simulink model "Orbit_SRP"  (R2021b)
settings: Solver=VariableStepAuto  StartTime=0.0  StopTime=SimTime  MaxStep=1e-2  RelTol=1e-13
values from neighbouring files (symbols this model uses):
  a = 8.6251e+06    (= 8625100)    [Lab7.m]    (also in Lab_7.m = 42164; car2kep.m = -(mu/(2*E)))
  e = 0.1195    [Lab7.m]    (also in Lab_7.m = 0; car2kep.m = 1/mu * [((v_norm)^2 - (mu/r_norm)).*r - (dot(r, v).*v)])
  i = acos(h_z/h_norm)    [car2kep.m]
  mu = 398600    [Lab_7.m]
undefined symbols (not defined in the file or in its folder): A_BN, theta_0
libraries: simulink_extras x1
settings Model: Creator=adity  LastModifiedBy=adity

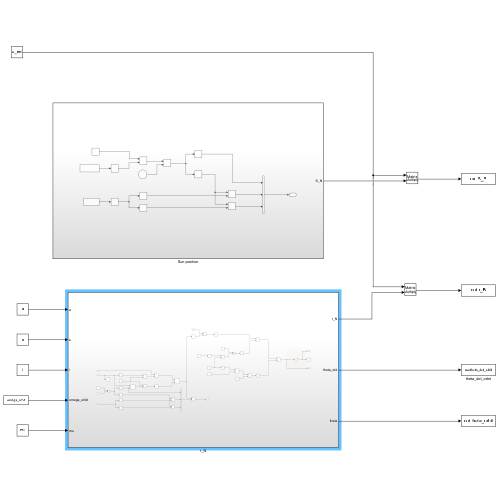
[thumbnail: Simulink's stored preview of the top-level diagram]
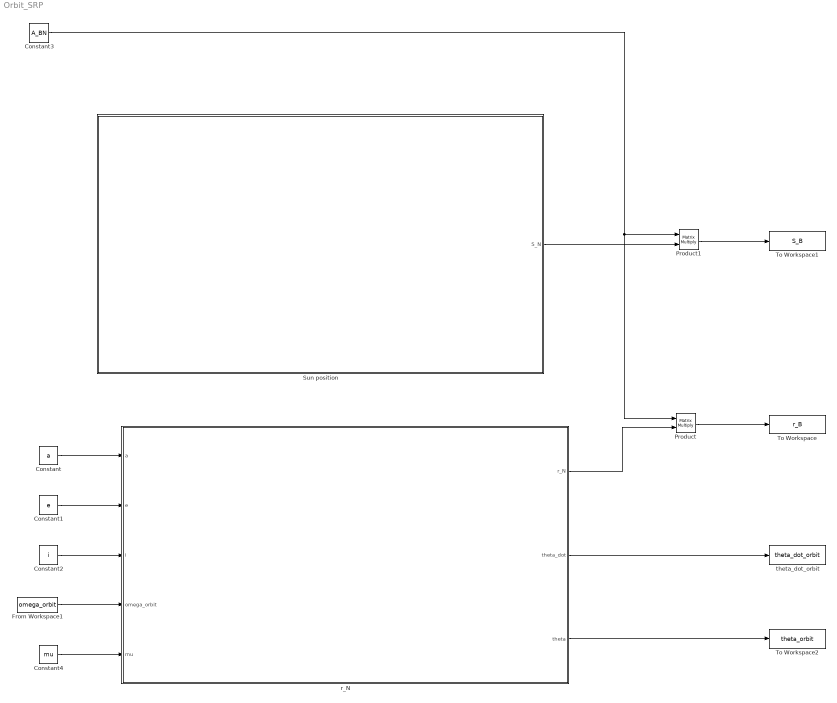
== system Orbit_SRP ==
  Constant : Constant  Value=a
  Constant1 : Constant  Value=e
  Constant2 : Constant  Value=i
  Constant3 : Constant  Value=A_BN
  Constant4 : Constant  Value=mu
  From Workspace1 : FromWorkspace  VariableName=omega_orbit
  Product : Product  Multiplication=Matrix(*)
  Product1 : Product  Multiplication=Matrix(*)
  Sun position : Subsystem
  To Workspace : ToWorkspace  VariableName=r_B  SaveFormat=Timeseries  SampleTime=-1
  To Workspace1 : ToWorkspace  VariableName=S_B  SaveFormat=Timeseries  SampleTime=-1
  To Workspace2 : ToWorkspace  VariableName=theta_orbit  SaveFormat=Timeseries  SampleTime=-1
  r_N : Subsystem
  theta_dot_orbit : ToWorkspace  VariableName=theta_dot_orbit  SaveFormat=Timeseries  SampleTime=-1
  wires:
  Constant/1 -> r_N/1(a)
  Constant1/1 -> r_N/2(e)
  Constant2/1 -> r_N/3(i)
  From Workspace1/1 -> r_N/4(omega_orbit)
  Constant4/1 -> r_N/5(mu)
  Constant3/1 -> Product/1, Product1/1
  r_N/1(r_N) -> Product/2
  Product/1 -> To Workspace/1
  r_N/2(theta_dot) -> theta_dot_orbit/1
  r_N/3(theta) -> To Workspace2/1
  Sun position/1(S_N) -> Product1/2
  Product1/1 -> To Workspace1/1

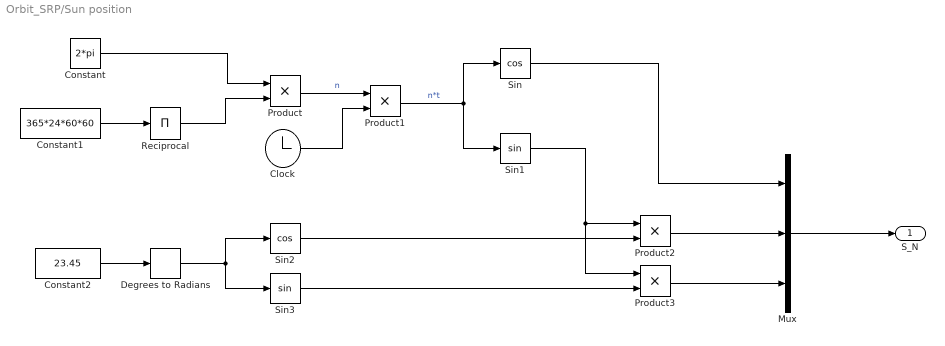
== system Orbit_SRP/Sun position ==
  Clock : Clock
  Constant : Constant  Value=2*pi
  Constant1 : Constant  Value=365*24*60*60
  Constant2 : Constant  Value=23.45
  Degrees to Radians : simulink_extras/Transformations/Degrees to Radians
  Mux : Mux  Inputs=3
  Product{,1..3} (4 alike) : Product
  Reciprocal : Product  Inputs=1
  Sin : Trigonometry  Operator=cos
  Sin1 : Trigonometry
  Sin2 : Trigonometry  Operator=cos
  Sin3 : Trigonometry
  S_N : Outport
  wires:
  Mux/1 -> S_N/1
  Constant1/1 -> Reciprocal/1
  Reciprocal/1 -> Product/2
  Constant/1 -> Product/1
  Product1/1 -> Sin/1, Sin1/1  "n*t"
  Product/1 -> Product1/1  "n"
  Clock/1 -> Product1/2
  Constant2/1 -> Degrees to Radians/1
  Sin/1 -> Mux/1
  Sin1/1 -> Product3/1, Product2/1
  Sin2/1 -> Product2/2
  Product2/1 -> Mux/2
  Sin3/1 -> Product3/2
  Product3/1 -> Mux/3
  Degrees to Radians/1 -> Sin3/1, Sin2/1

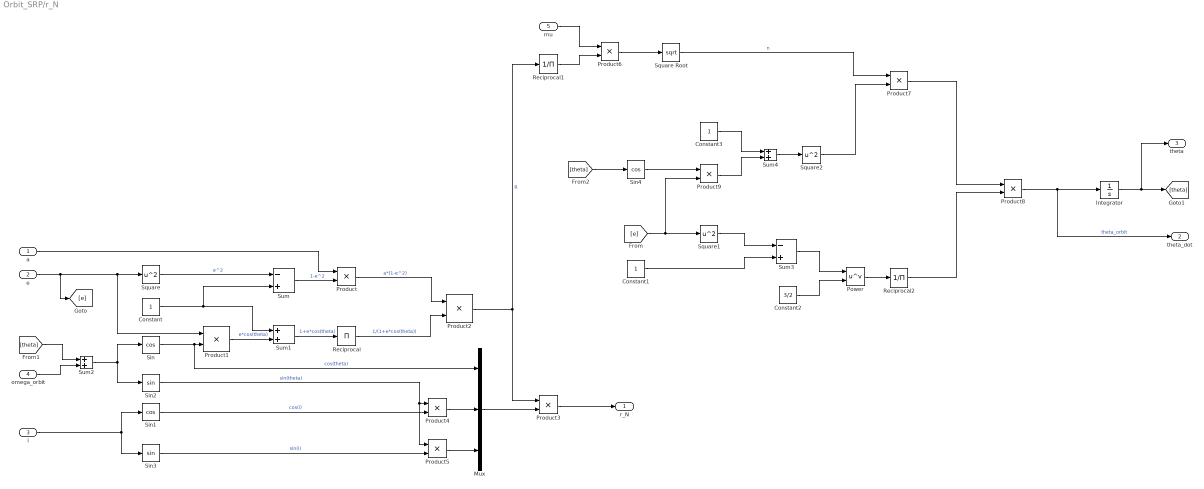
== system Orbit_SRP/r_N ==
  a : Inport
  e : Inport  Port=2
  i : Inport  Port=3
  omega_orbit : Inport  Port=4
  mu : Inport  Port=5
  Constant : Constant
  Constant1 : Constant
  Constant2 : Constant  Value=3/2
  Constant3 : Constant
  Integrator : Integrator  InitialCondition=theta_0
  Mux : Mux  Inputs=3
  Power : Math  Operator=pow  SaturateOnIntegerOverflow=on
  Product{,1..9} (10 alike) : Product
  Reciprocal : Product  Inputs=1
  Reciprocal1 : Product  Inputs=/
  Reciprocal2 : Product  Inputs=/
  Sin : Trigonometry  Operator=cos
  Sin1 : Trigonometry  Operator=cos
  Sin2 : Trigonometry
  Sin3 : Trigonometry
  Sin4 : Trigonometry  Operator=cos
  Square : Math  Operator=square  SaturateOnIntegerOverflow=on
  Square Root : Sqrt  SaturateOnIntegerOverflow=on
  Square1 : Math  Operator=square  SaturateOnIntegerOverflow=on
  Square2 : Math  Operator=square  SaturateOnIntegerOverflow=on
  Sum : Sum  Inputs=-+
  Sum1 : Sum
  Sum2 : Sum
  Sum3 : Sum  Inputs=-+
  Sum4 : Sum
  r_N : Outport
  theta_dot : Outport  Port=2
  theta : Outport  Port=3
  wires:
  e/1 -> [e], Square/1, Product1/1
  Square/1 -> Sum/1  "e^2"
  Constant/1 -> Sum1/1, Sum/2
  Sum/1 -> Product/2  "1-e^2"
  a/1 -> Product/1
  Sin/1 -> Mux/1, Product1/2  "cos(theta)"
  Product1/1 -> Sum1/2  "e*cos(theta)"
  Sum1/1 -> Reciprocal/1  "1+e*cos(theta)"
  Product/1 -> Product2/1  "a*(1-e^2)"
  Reciprocal/1 -> Product2/2  "1/(1+e*cos(theta))"
  i/1 -> Sin1/1, Sin3/1
  Product5/1 -> Mux/3
  Product4/1 -> Mux/2
  Product2/1 -> Reciprocal1/1, Product3/1  "R"
  Mux/1 -> Product3/2
  Product3/1 -> r_N/1
  Sin1/1 -> Product4/2  "cos(i)"
  Sin2/1 -> Product5/1, Product4/1  "sin(theta)"
  Sin3/1 -> Product5/2  "sin(i)"
  omega_orbit/1 -> Sum2/2
  Sum2/1 -> Sin2/1, Sin/1
  [theta] -> Sum2/1
  Product6/1 -> Square Root/1
  Reciprocal1/1 -> Product6/2
  mu/1 -> Product6/1
  [e] -> Square1/1, Product9/2
  Constant1/1 -> Sum3/2
  Square1/1 -> Sum3/1
  Sum3/1 -> Power/1
  Constant2/1 -> Power/2
  Square Root/1 -> Product7/1  "n"
  Power/1 -> Reciprocal2/1
  Product7/1 -> Product8/1
  Reciprocal2/1 -> Product8/2
  Product8/1 -> Integrator/1, theta_dot/1  "theta_orbit"
  Integrator/1 -> [theta], theta/1
  [theta] -> Sin4/1
  Sin4/1 -> Product9/1
  Constant3/1 -> Sum4/1
  Product9/1 -> Sum4/2
  Sum4/1 -> Square2/1
  Square2/1 -> Product7/2
